simulink model "s32ze_model_pil_block_simulink_r52"  (R2024a)
settings: Solver=FixedStepDiscrete  StartTime=0.0  StopTime=10  FixedStep=T  RelTol=1e-3
PreLoadFcn:
  | % NXP_MBDT_S32ZE callback: DO NOT REMOVE
  | mbd_s32ze.common.nxp.model_callbacks.preLoadFcn();
PostLoadFcn:
  | Increment = Simulink.Parameter;
  | Increment.DataType = 'uint8';
  | Increment.CoderInfo.StorageClass = 'SimulinkGlobal';
  | Increment.Value = 1;
  | 
  | SilCounterBus = Simulink.Bus;
  | SilCounterBus.Description = 'This bus contains counter inputs';
  | 
  | e1 = Simulink.BusElement;
  | e1.DataType = 'boolean';
  | e1.Name = 'ticks_to_count';
  | 
  | e2 = Simulink.BusElement;
  | e2.DataType = 'boolean';
  | e2.Name = 'reset';
  | 
  | SilCounterBus.Elements = [e1 e2];
  | clear e1 e2
  | 
  | % Step size
  | T=0.1;
  | 
  | % Input values
  | ticks_to_count.time = (0:100)'*T;
  | ticks_to_count.signals.values = boolean((floor( (0:100)/2)==(0:100)/2)');
  | ticks_to_count.signals.dimensions = 1;
  | 
  | reset.time = (0:100)'*T;
  | reset_values = boolean(zeros(101,1)); reset_values(20)=true;
  | reset.signals.values = reset_values;
  | clear reset_values
  | reset.signals.dimensions = 1;
  | % NXP_MBDT_S32ZE callback: DO NOT REMOVE
  | mbd_s32ze.common.nxp.model_callbacks.postLoadFcn();
InitFcn:
  | % NXP_MBDT_S32ZE callback: DO NOT REMOVE
  | mbd_s32ze.common.nxp.model_callbacks.initFcn();
Description:
  | R52 Mathworks Model PIL Block EBT
  | 
  | 
  | 
  |         R52 Mathworks Model PIL Block EBT
  |         <a href="matlab:open(fullfile(mbd_find_s32ze_root(),'S32ZE_Examples\r52\pil\s32ze_model_pil_block\model_pil_block_simulink_r52.slx'))">Open Example
  |         The model_pil_block_simulink_r52.slx example illustrates the Reference Model PIL (Processor-in-the-Loop) simulation.
  | 
  |             This example shows you how to use Embedded Coder® Support Package for ARM Cortex-R™ Processors for code verification and validation using PIL.
  | 
  |             Note: the initialization settings for the components used in this example represent just a default EB Tresos available configuration.Users can change the configuration of the application to fit special requirements.
  | 
  |         Toolchain Supported
  | 
  | 
  |                 S32 Design Studio v3.5.13
  | 
  | 
  |         Required Hardware
  | 
  | 
  |                 Personal Computer
  | 
  |                 S32Z2xx/S32E2xx
  | 
  |                 12V Power Supply
  | 
  |                 Micro USB cable
  | 
  |                 S32 Debugger probe
  | 
  | 
  |         Prepare the Demo
  | 
  | 
  |                 Open the model and select the processor package. This model is configured for the S32E2xx-bga975 hardware package. If you would like to change the processor package, please follow the steps described in the Customization Options section.
  | 
  |                 Connect the S32 Debugger probe to the J129 JTAG pin connector on the EVB.
  | 
  |                 Open the Hardware Settings of the model, go to Hardware Implementation -> Target hardware resources -> PIL tab.
  | 
  |                 For the Serial Port option, type the COM Port as identified inside Device Manager under the Ports tab.
  | 
  |                 UART default configuration is using the LINFLEXD instance 9 which is also used for serial boot on S32E27X-DC4 EVB. Disable the BootROM to be able to use the serial.
  | 
  | 
  |         Running the Demo
  | 
  | 
  |                 To validate this example, follow the steps from Code Verification and Validation with PIL page, <a href="https://www.mathworks.com/help/supportpkg/armcortexm/ref/code-verification-and-validation-with-pil-and-external-mode.html">Task 2 - Verify referenced model code using PIL
  | 
  |                 For starting the PIL simulation open the SIL/PIL Manager from the Apps tab.
  | 
  |                 From the SIL/PIL Manager App set the System Under Test to Model blocks in SIL/PIL mode.
  | 
  |                 Press the Run Verification button.
  | 
  | 
  |         Customization Options
  | 
  | 
  |                 How to change the processor package - visit section 6.8 of <a href="matlab:web(fullfile(mbd_find_s32ze_root(), 'mbdtbx_s32ze', 'help', 'release_notes.html'), '-browser')">Model_Based_Design_Toolbox_S32ZE_Series_Release_Notes
  | 
  |                 How to create a configuration project for a custom board - visit section 6.6 of <a href="matlab:web(fullfile(mbd_find_s32ze_root(), 'mbdtbx_s32ze', 'help', 'release_notes.html'), '-browser')">Model_Based_Design_Toolbox_S32ZE_Series_Release_Notes
  | 
  |                 For S32Z and S32E Design Tools and Files, please visit <a href="https://www.nxp.com/products/processors-and-microcontrollers/s32-automotive-platform/s32z-and-s32e-real-time-processors:S32Z-E-REAL-TIME-PROCESSORS">S32ZE Microcontrollers
settings Model: DataDictionary=s32ze_model_pil_block_simulink_r52.sldd  FPTRunName=Active  SILPILSystemUnderTest=refmodels  Creator=The MathWorks, Inc.  LastModifiedBy=nxg00842
settings SolverCC: AlgebraicLoopSolver=TrustRegion
settings DataIOCC: SaveFormat=StructureWithTime  SaveOutput=off  SaveTime=off  SignalLoggingName=logsOut
settings OptimizationCC: UseDivisionForNetSlopeComputation=UseDivisionForReciprocalsOfIntegersOnly  EnhancedBackFolding=on  BooleansAsBitfields=on  PassReuseOutputArgsAs=Individual arguments  ExpressionDepthLimit=2147483647  StateBitsets=on  DataBitsets=on  ZeroExternalMemoryAtStartup=off  ZeroInternalMemoryAtStartup=off  NoFixptDivByZeroProtection=on  EfficientFloat2IntCast=on  LifeSpan=1  MaxStackSize=64  SimCompilerOptimization=on  EfficientTunableParamExpr=on
settings DebuggingCC: ReadBeforeWriteMsg=DisableAll  WriteAfterWriteMsg=DisableAll  WriteAfterReadMsg=DisableAll  UnderspecifiedInitializationDetection=Classic  CheckExecutionContextPreStartOutputMsg=on  FcnCallInpInsideContextMsg=warning  UnconnectedInputMsg=warning  UnconnectedOutputMsg=warning  UnconnectedLineMsg=warning  UniqueDataStoreMsg=error  AllowSymbolicDim=off  ModelReferenceSymbolNameMessage=none  StateNameClashWarn=warning  StrictBusMsg=ErrorOnBusTreatedAsVector  SFUnexpectedBacktrackingDiag=warning  SFNoUnconditionalDefaultTransitionDiag=warning  SFExecutionAtInitializationDiag=none  ArithmeticOperatorsInVariantConditions=warning
settings HardwareCC: ProdBitPerPointer=32  ProdBitPerSizeT=32  ProdBitPerPtrDiffT=32  ProdLargestAtomicInteger=Long  ProdLargestAtomicFloat=Double  ProdWordSize=32  ProdHWDeviceType=ARM Compatible->ARM Cortex  TargetHWDeviceType=Generic->32-bit Embedded Processor
settings ModelReferenceCC: EnableRefExpFcnMdlSchedulingChecks=on  CheckModelReferenceTargetMessage=none  PropagateSignalLabelsOutOfModel=off
settings SFSimCC: SimUseLocalCustomCode=off  MATLABDynamicMemAlloc=off  CustomCodeUndefinedFunction=UseInterfaceOnly
settings RTWCC: Description=Embedded Coder  SystemTargetFile=ert.tlc  HardwareBoard=NXP S32ZE2xx  TemplateMakefile=ert_default_tmf  GenerateReport=on  RTWVerbose=off  RTWUseLocalCustomCode=off  Toolchain=NXP S32 Design Studio GCC (S32ZE)  BuildConfiguration=Debug  IncludeHyperlinkInReport=on  CodeExecutionProfiling=on  CodeProfilingInstrumentation=coarse  GenerateTraceInfo=on  GenerateTraceReport=on  GenerateTraceReportSl=on  GenerateTraceReportSf=on  GenerateTraceReportEml=on  GenerateWebview=on  GenerateCodeMetricsReport=on  GPUComputeCapability=3.5  DLArmComputeVersion=19.05
settings CodeAppCC: ForceParamTrailComments=on  IgnoreCustomStorageClasses=off  SimulinkDataObjDesc=on  CustomSymbolStrGlobalVar=rt$N$M  CustomSymbolStrType=$N$M  CustomSymbolStrFcn=$N$M$F  CustomSymbolStrMacro=$N$M  InsertBlockDesc=on  StateflowObjectComments=on  InternalIdentifier=Classic
settings ERTTargetCC: UtilityFuncGeneration=Shared location  MultiwordLength=2048  IncludeMdlTerminateFcn=off  CombineSignalStateStructs=on  SupportNonFinite=off  SupportComplex=off  SupportNonInlinedSFcns=on  ExtModeTransport=1  ExtModeMexFile=ext_serial_win32_comm  ERTSrcFileBannerTemplate=mbd_s32ze_ert_code_template.cgt  ERTHdrFileBannerTemplate=mbd_s32ze_ert_code_template.cgt  ERTDataSrcFileTemplate=mbd_s32ze_ert_code_template.cgt  ERTDataHdrFileTemplate=mbd_s32ze_ert_code_template.cgt  ERTFilePackagingFormat=CompactWithDataFile  ConvertIfToSwitch=off  SuppressUnreachableDefaultCases=off
settings ConfigComp: CovMetricSettings=dw  CovSaveCumulativeToWorkspaceVar=on  CovSaveSingleToWorkspaceVar=on  CovExternalEMLEnable=off  CovSFcnEnable=off

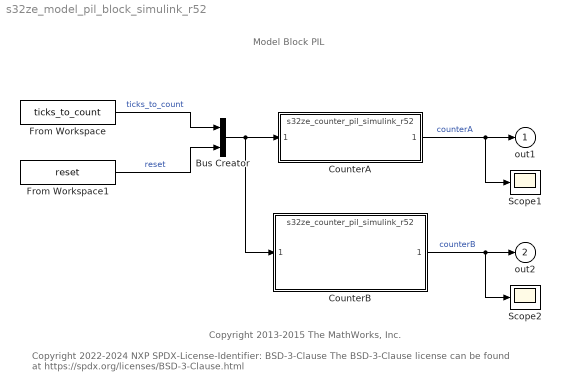
== system s32ze_model_pil_block_simulink_r52 ==
  note: Copyright 2013-2015 The MathWorks, Inc.
  note: Model Block PIL
  note: Copyright 2022-2024 NXP
      |
      | SPDX-License-Identifier: BSD-3-Clause
      | The BSD-3-Clause license can be found at https://spdx.org/licenses/BSD-3-Clause.html
  Bus Creator : BusCreator  Inputs='ticks_to_count','reset'  OutDataTypeStr=Bus: SilCounterBus  NonVirtualBus=on
  CounterA : ModelReference  ModelNameDialog=s32ze_counter_pil_simulink_r52.slx  UsingDefaultArgumentValue=0,0  SimulationMode=Processor-in-the-loop (PIL)  ModelReferenceVersion=23
  CounterB : ModelReference  ModelNameDialog=s32ze_counter_pil_simulink_r52.slx  UsingDefaultArgumentValue=0,0  SimulationMode=Normal  ModelReferenceVersion=23
  From Workspace : FromWorkspace  VariableName=ticks_to_count  SampleTime=T
  From Workspace1 : FromWorkspace  VariableName=reset  SampleTime=T
  Scope1 : Scope
  Scope2 : Scope
  out1 : Outport  VectorParamsAs1DForOutWhenUnconnected=off
  out2 : Outport  Port=2  VectorParamsAs1DForOutWhenUnconnected=off
  wires:
  CounterA/1 -> Scope1/1, out1/1  "counterA"
  Bus Creator/1 -> CounterA/1, CounterB/1
  From Workspace/1 -> Bus Creator/1  "ticks_to_count"
  From Workspace1/1 -> Bus Creator/2  "reset"
  CounterB/1 -> out2/1, Scope2/1  "counterB"
